simulink model "Body_Khoo"  (Simulink 6.4)
settings: Solver=ode45  StartTime=0.0  StopTime=10.0  RelTol=1e-3
values from neighbouring files (symbols this model uses):
  CvCO2IC = 0.5116    [Body_Khoo_IC.m]    (also in Gas_Exchange_IC.m; Respiratory_IC.m = 0.5247)
  CvO2IC = 0.1672    [Body_Khoo_IC.m]    (also in Gas_Exchange_IC.m; Respiratory_IC.m = 0.1639)
  MRCO2 = 0.0033    [Body_Khoo_IC.m]    (also in Gas_Exchange_IC.m; Respiratory_IC.m)
  MRO2 = 0.0038    [Body_Khoo_IC.m]    (also in Gas_Exchange_IC.m; Respiratory_IC.m)
  VTCO2 = 15    [Body_Khoo_IC.m]    (also in Gas_Exchange_IC.m; Respiratory_IC.m)
  VTO2 = 6    [Body_Khoo_IC.m]    (also in Gas_Exchange_IC.m; Respiratory_IC.m)
settings Model: LastModifiedBy=CLM
settings OptimizationCC: BlockReduction=off  BooleanDataType=off
settings DebuggingCC: SolverPrmCheckMsg=none  StrictBusMsg=None
settings HardwareCC: TargetUnknown=on

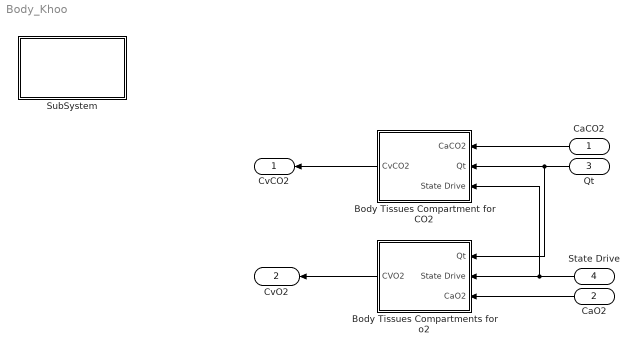
== system Body_Khoo ==
  CaCO2 : Inport  Orientation=left
  CaO2 : Inport  Orientation=left  Port=2
  "Qt " : Inport  Orientation=left  Port=3
  State Drive : Inport  Orientation=left  Port=4
  Body Tissues Compartment for CO2 : Subsystem  Orientation=left
  Body Tissues Compartments for o2 : Subsystem  Orientation=left
  SubSystem : Subsystem
      settings: OpenFcn=Body_Khoo_IC
      mask Display: disp('"double click here"\n to load \nBody_Khoo \ninitial values');
  CvCO2 : Outport  Orientation=left
  CvO2 : Outport  Orientation=left  Port=2
  wires:
  "Qt "/1 -> Body Tissues Compartment for CO2/2(Qt), Body Tissues Compartments for o2/1("Qt ")
  Body Tissues Compartments for o2/1(CVO2) -> CvO2/1
  Body Tissues Compartment for CO2/1(CvCO2) -> CvCO2/1
  CaO2/1 -> Body Tissues Compartments for o2/3(CaO2)
  CaCO2/1 -> Body Tissues Compartment for CO2/1(CaCO2)
  State Drive/1 -> Body Tissues Compartment for CO2/3(State Drive), Body Tissues Compartments for o2/2(State Drive)

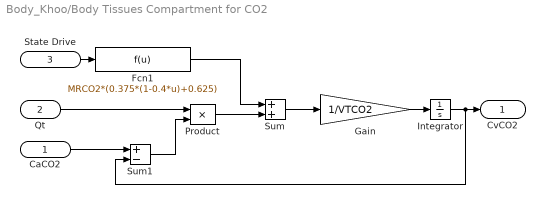
== system Body_Khoo/Body Tissues Compartment for CO2 ==
  CaCO2 : Inport
  Qt : Inport  Port=2
  State Drive : Inport  Port=3
  Fcn1 : Fcn  Expr=MRCO2*(0.375*(1-0.4*u)+0.625)
  Gain : Gain  Gain=1/VTCO2  SaturateOnIntegerOverflow=on
  Integrator : Integrator  InitialCondition=CvCO2IC
  Product : Product  SaturateOnIntegerOverflow=on  RndMeth=Zero  InputSameDT=on
  Sum : Sum  SaturateOnIntegerOverflow=on  InputSameDT=on
  Sum1 : Sum  Inputs=+-  SaturateOnIntegerOverflow=on  InputSameDT=on
  CvCO2 : Outport
  wires:
  Fcn1/1 -> Sum/1
  State Drive/1 -> Fcn1/1
  Qt/1 -> Product/1
  CaCO2/1 -> Sum1/1
  Sum1/1 -> Product/2
  Product/1 -> Sum/2
  Sum/1 -> Gain/1
  Gain/1 -> Integrator/1
  Integrator/1 -> CvCO2/1, Sum1/2

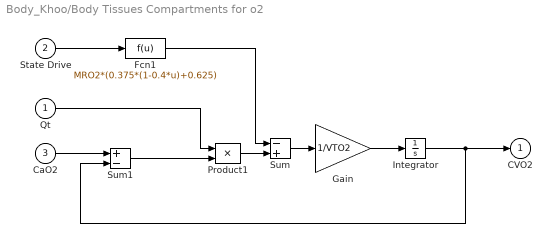
== system Body_Khoo/Body Tissues Compartments for o2 ==
  "Qt " : Inport
  State Drive : Inport  Port=2
  CaO2 : Inport  Port=3
  Fcn1 : Fcn  Expr=MRO2*(0.375*(1-0.4*u)+0.625)
  Gain : Gain  Gain=1/VTO2  SaturateOnIntegerOverflow=on
  Integrator : Integrator  InitialCondition=CvO2IC
  Product1 : Product  SaturateOnIntegerOverflow=on  RndMeth=Zero  InputSameDT=on
  Sum : Sum  Inputs=-+  SaturateOnIntegerOverflow=on  InputSameDT=on
  Sum1 : Sum  Inputs=+-  SaturateOnIntegerOverflow=on  InputSameDT=on
  CVO2 : Outport
  wires:
  Fcn1/1 -> Sum/1
  State Drive/1 -> Fcn1/1
  "Qt "/1 -> Product1/1
  Sum1/1 -> Product1/2
  CaO2/1 -> Sum1/1
  Integrator/1 -> CVO2/1, Sum1/2
  Product1/1 -> Sum/2
  Sum/1 -> Gain/1
  Gain/1 -> Integrator/1

== system Body_Khoo/SubSystem ==
